simulink subsystem "sistema_LTI_aumentado"  (R2023b)
settings: Solver=VariableStepAuto  StartTime=0.0  StopTime=10.0  RelTol=1e-3
values from neighbouring files (symbols this model uses):
  b_eq = b_m + b_l/(r^2)    (= 2.19444444444e-05)    [constantes.m]    (also in test_polos_PID.m = b_m + b_l_nominal/(r^2))
  C_ts = 0.818    [constantes.m]
  J_eq = J_m + J_l/(r^2)    (= 1.97847222222e-05)    [constantes.m]    (also in test_polos_PID.m = J_m + J_l/(r^2))
  k_l = g*(m*l_cm + m_l*l_l)    (= 2.4516625)    [constantes.m]
  lambda_m = 0.016    [constantes.m]
  Ld = 6.6e-3    (= 0.0066)    [constantes.m]
  Lq = 5.8e-3    (= 0.0058)    [constantes.m]
  P_p = 3    [constantes.m]
  r = 120    [constantes.m]
  R_sREF = 1.02    [constantes.m]
  R_ts_amb = 146.7    [constantes.m]
  T_s_inicial = 40    [constantes.m]
settings Model: Creator=nahue  LastModifiedBy=nahue

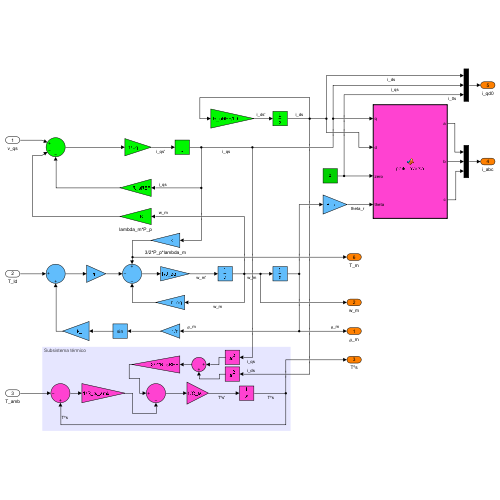
[thumbnail: Simulink's stored preview of the top-level diagram]
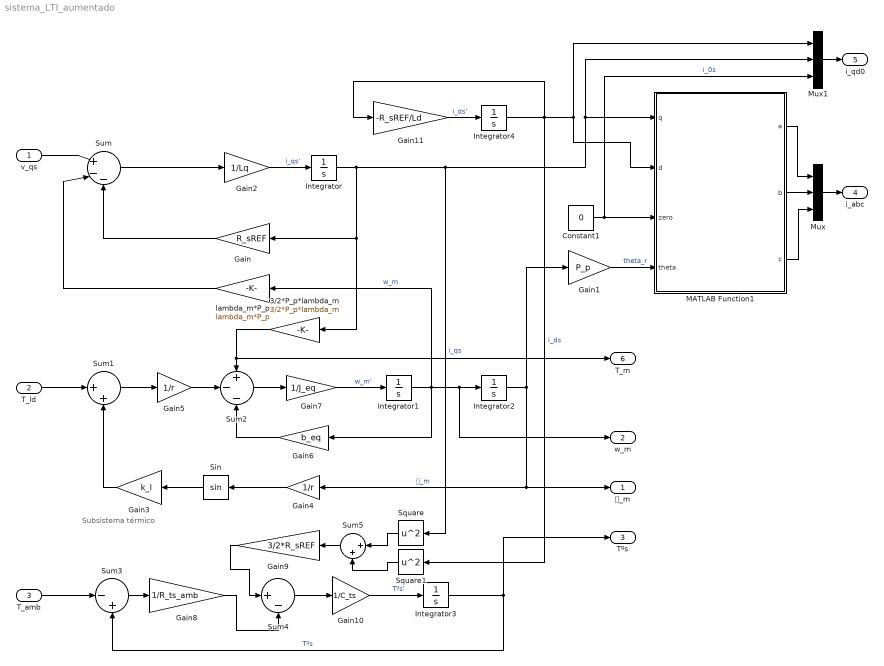
== system sistema_LTI_aumentado ==
  note: Subsistema térmico
  v_qs : Inport
  T_ld : Inport  Port=2
  T_amb : Inport  Port=3
  3/2*P_p*lambda_m : Gain  Gain=3/2*P_p*lambda_m
  Constant1 : Constant  Value=0
  Gain : Gain  Gain=R_sREF
  Gain1 : Gain  Gain=P_p
  Gain10 : Gain  Gain=1/C_ts
  Gain11 : Gain  Gain=-R_sREF/Ld
  Gain2 : Gain  Gain=1/Lq
  Gain3 : Gain  Gain=k_l
  Gain4 : Gain  Gain=1/r
  Gain5 : Gain  Gain=1/r
  Gain6 : Gain  Gain=b_eq
  Gain7 : Gain  Gain=1/J_eq
  Gain8 : Gain  Gain=1/R_ts_amb
  Gain9 : Gain  Gain=3/2*R_sREF
  Integrator{,1..2,4} (4 alike) : Integrator
  Integrator3 : Integrator  InitialCondition=T_s_inicial
  MATLAB Function1 : MATLAB Function  TreatAsAtomicUnit=on
  Mux : Mux  Inputs=3
  Mux1 : Mux  Inputs=3
  Sin : Trigonometry
  Square : Math  Operator=square
  Square1 : Math  Operator=square
  Sum : Sum  Inputs=|+--
  Sum1 : Sum  Inputs=|++
  Sum2 : Sum  Inputs=+--
  Sum3 : Sum  Inputs=|-+
  Sum4 : Sum  Inputs=|+-
  Sum5 : Sum  Inputs=|++
  lambda_m*P_p : Gain  Gain=lambda_m*P_p
  𝜃_m : Outport
  w_m : Outport  Port=2
  Tºs : Outport  Port=3
  i_abc : Outport  Port=4
  i_qd0 : Outport  Port=5
  T_m : Outport  Port=6
  wires:
  Gain/1 -> Sum/3
  lambda_m*P_p/1 -> Sum/2
  Sum/1 -> Gain2/1
  Gain2/1 -> Integrator/1  "i_qs'"
  Integrator/1 -> 3/2*P_p*lambda_m/1, Gain/1, Square/1, Mux1/2, MATLAB Function1/1(q)  "i_qs"
  T_ld/1 -> Sum1/1
  Gain3/1 -> Sum1/2
  Sin/1 -> Gain3/1
  Gain4/1 -> Sin/1
  Sum1/1 -> Gain5/1
  Gain5/1 -> Sum2/2
  3/2*P_p*lambda_m/1 -> Sum2/1, T_m/1
  Gain6/1 -> Sum2/3
  Sum2/1 -> Gain7/1
  Gain7/1 -> Integrator1/1  "w_m'"
  Integrator1/1 -> w_m/1, Integrator2/1, Gain6/1, lambda_m*P_p/1  "w_m"
  Integrator2/1 -> Gain1/1, 𝜃_m/1, Gain4/1  "𝜃_m"
  Gain1/1 -> MATLAB Function1/4(theta)  "theta_r"
  Constant1/1 -> Mux1/3, MATLAB Function1/3(zero)  "i_0s"
  T_amb/1 -> Sum3/1
  Sum3/1 -> Gain8/1
  Gain8/1 -> Sum4/2
  Gain9/1 -> Sum4/1
  Square/1 -> Sum5/1
  Sum4/1 -> Gain10/1
  Gain10/1 -> Integrator3/1  "Tºs'"
  Integrator3/1 -> Sum3/2, Tºs/1  "Tºs"
  MATLAB Function1/1(a) -> Mux/1
  MATLAB Function1/2(b) -> Mux/2
  MATLAB Function1/3(c) -> Mux/3
  Mux/1 -> i_abc/1
  Gain11/1 -> Integrator4/1  "i_ds'"
  Integrator4/1 -> Mux1/1, MATLAB Function1/2(d), Gain11/1, Square1/1  "i_ds"
  Mux1/1 -> i_qd0/1
  Square1/1 -> Sum5/2
  Sum5/1 -> Gain9/1
  v_qs/1 -> Sum/1

== matlab function sistema_LTI_aumentado/MATLAB Function1 ==
  data: q input; d input; a output; zero input; theta input; b output; c output
function [a, b, c] = park_inversa(q, d, zero, theta)
    % Transformación de Park Inversa
    % Entradas:
    %   d, q, z: Coordenadas en el marco rotatorio
    %   theta: Ángulo en radianes
    % Salidas:
    %   a, b, c: Valores trifásicos reconstruidos
    
    % Constantes
    alpha = 2 * pi / 3; % Desplazamiento angular entre fases
    
    % Cálculo de valores trifásicos
    a = q * cos(theta) + d * sin(theta) + zero;
    b = q * cos(theta - alpha) + d * sin(theta - alpha) + zero;
    c = q * cos(theta + alpha) + d * sin(theta + alpha) + zero;
end
